simulink model "sim_finale_1"  (R2024a)
settings: Solver=FixedStepAuto  StartTime=0.0  StopTime=40  FixedStep=0.001  RelTol=1e-3
undefined symbols (not defined in the file): A_p, A_y, aero_variabile_con_M, Attitude_0, Attitude_riferimento, b, B_p, B_pz, B_y, B_yz, C_A, C_l, C_m_alpha, C_N_alpha, C_p, C_y, conv_cost_distE, conv_cost_distN, conv_cost_eta, conv_cost_p, conv_cost_y, conv_cost_zeta, D_pz, D_yz, Env, F, G_wE, G_wN, G_xp, G_xy, I_sp, inertia_p, inertia_s, inertia_tot, L, m_p, m_s, m_tot, MIL, Moderate, P_p, P_y, R, r_cp_cm, r_nozzle_cm, S_rif, spinta_variabile, T_c, T_r, v_0, V_r, VelocitB_riferimento, w_0
libraries: cstblocks x16, simulink_extras x5, slpidlib x4, simulink x3, aerolibasang x3, aerolibwind2 x3, matrix_library x2, shared6dof x2, aerolibatmos2 x2, aerolibutil x1, aerolibanim x1
(part 2 of 2)

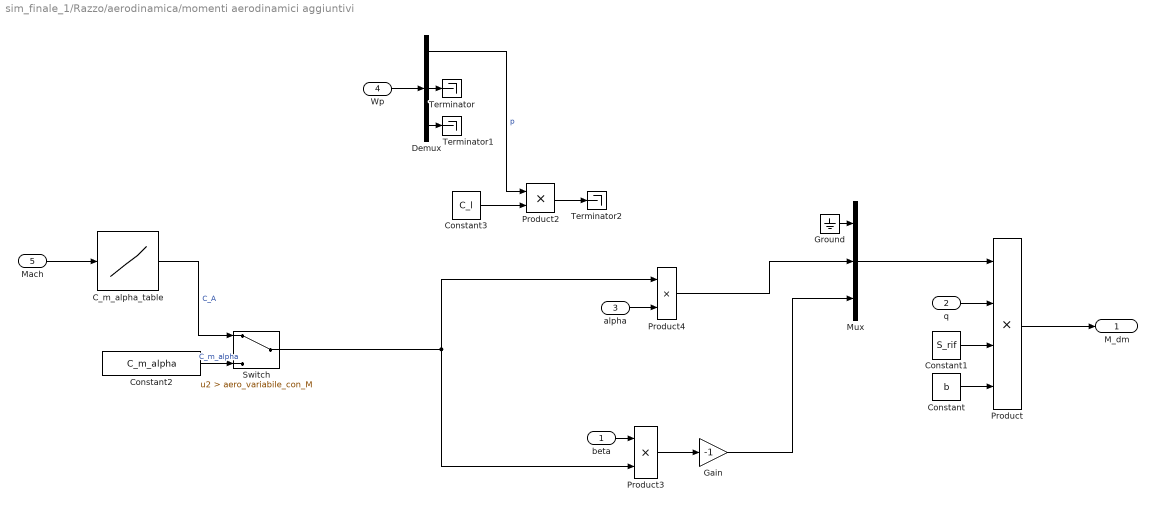
== system sim_finale_1/Razzo/aerodinamica/momenti aerodinamici aggiuntivi ==
  beta : Inport
  q : Inport  Port=2
  alpha : Inport  Port=3
  Wp : Inport  Port=4
  Mach : Inport  Port=5
  C_m_alpha_table : Lookup_n-D  NumberOfTableDimensions=1  BreakpointsForDimension1=[0;0.7;0.95;1.35;1.5;1.95;2.8;3;3.5;4;4.5;5]  Table=[1.75;2;2.05;2.2;2.25;2.5;3.4;3.45;3.6;4.05;4.15;5.15]  InternalRulePriority=Speed  RndMeth=Simplest
  Constant : Constant  Value=b
  Constant1 : Constant  Value=S_rif
  Constant2 : Constant  Value=C_m_alpha
  Constant3 : Constant  Value=C_l
  Demux : Demux  Outputs=3
  Gain : Gain  Gain=-1
  Ground : Ground
  Mux : Mux  Inputs=3
  Product : Product  Inputs=4
  Product2 : Product
  Product3 : Product
  Product4 : Product
  Switch : Switch  Criteria=u2 > Threshold  Threshold=aero_variabile_con_M  SaturateOnIntegerOverflow=off  InputSameDT=off
  Terminator : Terminator
  Terminator1 : Terminator
  Terminator2 : Terminator
  M_dm : Outport
  wires:
  Mux/1 -> Product/1
  Product/1 -> M_dm/1
  Wp/1 -> Demux/1
  Demux/1 -> Product2/1  "p"
  Constant3/1 -> Product2/2
  Product3/1 -> Gain/1
  Constant1/1 -> Product/3
  Constant/1 -> Product/4
  q/1 -> Product/2
  Gain/1 -> Mux/3
  Product4/1 -> Mux/2
  alpha/1 -> Product4/2
  beta/1 -> Product3/1
  Demux/2 -> Terminator/1
  Demux/3 -> Terminator1/1
  Product2/1 -> Terminator2/1
  Ground/1 -> Mux/1
  Switch/1 -> Product4/1, Product3/2
  Constant2/1 -> Switch/3  "C_m_alpha"
  C_m_alpha_table/1 -> Switch/1  "C_A"
  Mach/1 -> C_m_alpha_table/1

== system sim_finale_1/Razzo/massa/massa costante ==
  Constant : Constant  Value=m_tot
  Constant1 : Constant  Value=m_p
  Constant6 : Constant  Value=inertia_tot
  Ground : Ground
  I : Outport
  I_dot : Outport  Port=2
  m : Outport  Port=3
  tag scope: m_p=global
  wires:
  Constant/1 -> m/1
  Ground/1 -> I_dot/1
  Constant6/1 -> I/1
  Constant1/1 -> [m_p]

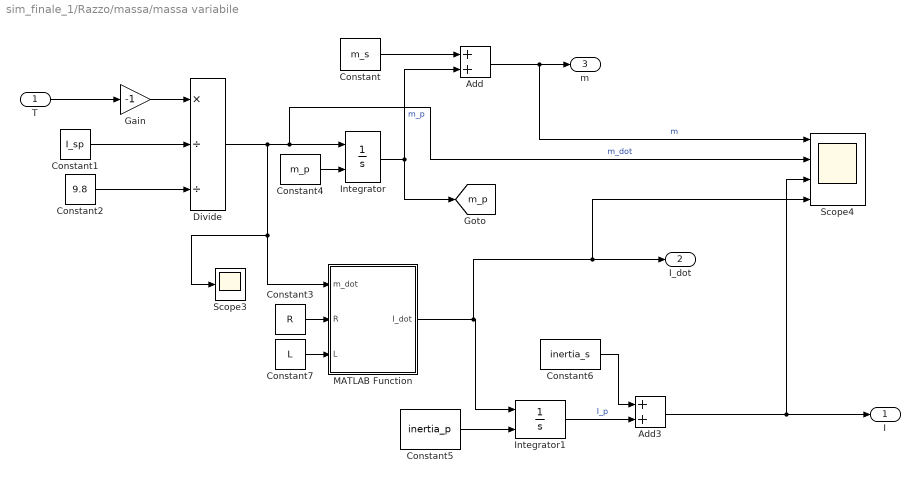
== system sim_finale_1/Razzo/massa/massa variabile ==
  T : Inport
  Add : Sum
  Add3 : Sum
  Constant : Constant  Value=m_s
  Constant1 : Constant  Value=I_sp
  Constant2 : Constant  Value=9.8
  Constant3 : Constant  Value=R
  Constant4 : Constant  Value=m_p
  Constant5 : Constant  Value=inertia_p
  Constant6 : Constant  Value=inertia_s
  Constant7 : Constant  Value=L
  Divide : Product  Inputs=*//
  Gain : Gain  Gain=-1
  Integrator : Integrator  InitialConditionSource=external  LimitOutput=on  LowerSaturationLimit=0
  Integrator1 : Integrator  InitialConditionSource=external  InitialCondition=inertia_p  LimitOutput=on  LowerSaturationLimit=zeros(3)
  MATLAB Function : MATLAB Function  TreatAsAtomicUnit=on
  Scope3 : Scope
  Scope4 : Scope  NumInputPorts=4
  I : Outport
  I_dot : Outport  Port=2
  m : Outport  Port=3
  tag scope: m_p=global
  wires:
  Constant1/1 -> Divide/2
  Constant7/1 -> MATLAB Function/3(L)
  Integrator/1 -> [m_p], Add/2  "m_p"
  Add3/1 -> I/1, Scope4/3
  Constant6/1 -> Add3/1
  Gain/1 -> Divide/1
  Constant4/1 -> Integrator/2
  Constant3/1 -> MATLAB Function/2(R)
  T/1 -> Gain/1
  Add/1 -> Scope4/1, m/1  "m"
  Constant5/1 -> Integrator1/2
  Constant2/1 -> Divide/3
  Constant/1 -> Add/1
  Divide/1 -> Scope3/1, MATLAB Function/1(m_dot), Scope4/2, Integrator/1  "m_dot"
  Integrator1/1 -> Add3/2  "I_p"
  MATLAB Function/1(I_dot) -> Scope4/4, I_dot/1, Integrator1/1

== system sim_finale_1/Variant Subsystem/meno reale/Ambiente ==
  BusElementIn : Inport  PortName=State  Element=Xe
  Atmosfera e gravità : Subsystem  Variant=on
  Demux : Demux  Outputs=3
  Scope : Scope  NumInputPorts=3
  Terminator : Terminator
  Terminator1 : Terminator
  Variant Subsystem : Subsystem  Variant=on
  Bus Element Out : Outport  PortName=Environment  Element=AirDensity
  BusElementOut : Outport  PortName=Environment  Element=SpeedOfSound
  BusElementOut1 : Outport  PortName=Environment  Element=Gravity
  BusElementOut2 : Outport  PortName=Environment  Element=Wind
  BusElementOut3 : Outport  PortName=Environment  Element=Temperature
  wires:
  Demux/1 -> Variant Subsystem/1(Heigh), Atmosfera e gravità/1(Height)  "h"
  Atmosfera e gravità/2(Speed of Sound) -> BusElementOut/1
  Atmosfera e gravità/4(Gravity) -> Scope/1, BusElementOut1/1
  Atmosfera e gravità/1(Temperature) -> BusElementOut3/1
  Variant Subsystem/1(WInd) -> Scope/3, BusElementOut2/1
  BusElementIn/1 -> Demux/1
  Demux/2 -> Terminator/1
  Demux/3 -> Terminator1/1
  Atmosfera e gravità/3(Air Density) -> Scope/2, Bus Element Out/1

== system sim_finale_1/Variant Subsystem/reale/Ambiente1 ==
  BusElementIn : Inport  PortName=State  Element=Xe
  BusElementIn1 : Inport  PortName=State  Element=DCM
  BusElementIn2 : Inport  PortName=State  Element=Vb
  Demux : Demux  Outputs=3
  Scope : Scope  NumInputPorts=3
  Subsystem : Subsystem
  Terminator : Terminator
  Terminator1 : Terminator
  Bus Element Out : Outport  PortName=Environment  Element=AirDensity
  BusElementOut : Outport  PortName=Environment  Element=SpeedOfSound
  BusElementOut1 : Outport  PortName=Environment  Element=Gravity
  BusElementOut2 : Outport  PortName=Environment  Element=Wind
  wires:
  Demux/1 -> Subsystem/3(Height)  "h"
  Subsystem/2(Speed of Sound) -> BusElementOut/1, Scope/3  "a"
  Subsystem/4(Gravity) -> BusElementOut1/1, Scope/1  "g"
  BusElementIn/1 -> Demux/1
  Demux/2 -> Terminator/1
  Demux/3 -> Terminator1/1
  Subsystem/3(Air Density) -> Bus Element Out/1, Scope/2  "rho"
  BusElementIn1/1 -> Subsystem/1(DCM)
  BusElementIn2/1 -> Subsystem/2(Vb)
  Subsystem/1(Wind) -> BusElementOut2/1

== system sim_finale_1/Razzo/Subsystem/Equazioni del moto/Eq. massa costante ==
  F_xyz : Inport
  M_xyz : Inport  Port=2
  6DOF (Euler Angles) : shared6dof/6DOF (Euler Angles)  units=Metric (MKS)  mtype=Fixed  rep=Euler Angles  xme_0=x_0  Vm_0=v_0  eul_0=Attitude_0  pm_0=w_0  mass_0=m_tot  mass_e=0.5  mass_f=2.0  inertia=inertia_tot  inertia_e=eye(3)  inertia_f=2*eye(3)  k_quat=1.0  vre_flag=on  abi_flag=on  aMode=0  xme_statename=''  Vm_statename=''  eul_statename=''  quat_statename=''  pm_statename=''  mass_statename=''
  Ve : Outport
  Xe : Outport  Port=2
  Attitude : Outport  Port=3
  DCM : Outport  Port=4
  Vb : Outport  Port=5
  Wb : Outport  Port=6
  Wb_dot : Outport  Port=7
  Ab : Outport  Port=8
  Ae : Outport  Port=9
  wires:
  6DOF (Euler Angles)/4 -> DCM/1
  F_xyz/1 -> 6DOF (Euler Angles)/1
  M_xyz/1 -> 6DOF (Euler Angles)/2
  6DOF (Euler Angles)/1 -> Ve/1
  6DOF (Euler Angles)/2 -> Xe/1
  6DOF (Euler Angles)/3 -> Attitude/1
  6DOF (Euler Angles)/5 -> Vb/1  "v_b"
  6DOF (Euler Angles)/6 -> Wb/1
  6DOF (Euler Angles)/7 -> Wb_dot/1
  6DOF (Euler Angles)/8 -> Ab/1
  6DOF (Euler Angles)/9 -> Ae/1

== system sim_finale_1/Razzo/Subsystem/Equazioni del moto/Eq. massa variabile ==
  F_xyz : Inport
  M_xyz : Inport  Port=2
  m : Inport  Port=3
  dI/dt : Inport  Port=4
  I : Inport  Port=5
  Custom Variable Mass 6DOF (Euler Angles) : shared6dof/6DOF (Euler Angles)  units=Metric (MKS)  mtype=Custom Variable  rep=Euler Angles  xme_0=x_0  Vm_0=v_0  eul_0=Attitude_0  pm_0=w_0  mass_0=1.0  mass_e=0.5  mass_f=2.0  inertia=eye(3)  inertia_e=eye(3)  inertia_f=2*eye(3)  k_quat=1.0  vre_flag=off  abi_flag=on  aMode=0  xme_statename=''  Vm_statename=''  eul_statename=''  quat_statename=''  pm_statename=''  mass_statename=''
      settings: LibrarySourceBlock=aerolib6dof2/Custom Variable Mass 6DOF (Euler Angles)
  Ve : Outport
  Xe : Outport  Port=2
  Attitude : Outport  Port=3
  DCM : Outport  Port=4
  Vb : Outport  Port=5
  Wb : Outport  Port=6
  Wb_dot : Outport  Port=7
  Ab : Outport  Port=8
  Ae : Outport  Port=9
  wires:
  F_xyz/1 -> Custom Variable Mass 6DOF (Euler Angles)/1
  M_xyz/1 -> Custom Variable Mass 6DOF (Euler Angles)/2
  m/1 -> Custom Variable Mass 6DOF (Euler Angles)/3
  dI/dt/1 -> Custom Variable Mass 6DOF (Euler Angles)/4
  I/1 -> Custom Variable Mass 6DOF (Euler Angles)/5
  Custom Variable Mass 6DOF (Euler Angles)/1 -> Ve/1
  Custom Variable Mass 6DOF (Euler Angles)/2 -> Xe/1
  Custom Variable Mass 6DOF (Euler Angles)/4 -> DCM/1
  Custom Variable Mass 6DOF (Euler Angles)/9 -> Ae/1
  Custom Variable Mass 6DOF (Euler Angles)/3 -> Attitude/1
  Custom Variable Mass 6DOF (Euler Angles)/5 -> Vb/1  "v_b"
  Custom Variable Mass 6DOF (Euler Angles)/6 -> Wb/1
  Custom Variable Mass 6DOF (Euler Angles)/8 -> Ab/1
  Custom Variable Mass 6DOF (Euler Angles)/7 -> Wb_dot/1

== system sim_finale_1/Razzo/aerodinamica/Calcolo F_a e M_a dovuto a F_a in X_a/C_A C_N_alpha ==
  Mach : Inport
  C_A C_N costanti : Subsystem  VariantControl=aero_variabile_con_M == false
  C_A e C_N variabili : Subsystem  VariantControl=aero_variabile_con_M == true
  C_A : Outport
  C_N_alpha : Outport  Port=2

== system sim_finale_1/Variant Subsystem/meno reale/Ambiente/Atmosfera e gravità ==
  Height : Inport
  Env costante : Subsystem  VariantControl="env_variabile  == false"
  Env variabile : Subsystem  VariantControl=env_variabile == true
  Temperature : Outport
  Speed of Sound : Outport  Port=2
  Air Density : Outport  Port=3
  Gravity : Outport  Port=4

== system sim_finale_1/Variant Subsystem/meno reale/Ambiente/Variant Subsystem ==
  note: 1) Add Subsystem or Model blocks as valid variant choices.
      | 2) You cannot connect blocks at this level. At simulation, connectivity is automatically
      | determined, based on the active variant and port name matching.
  Heigh : Inport
  cost Wind : Subsystem  VariantControl=dist_agg==false
  sin Wind : Subsystem  VariantControl=dist_agg==true
  WInd : Outport

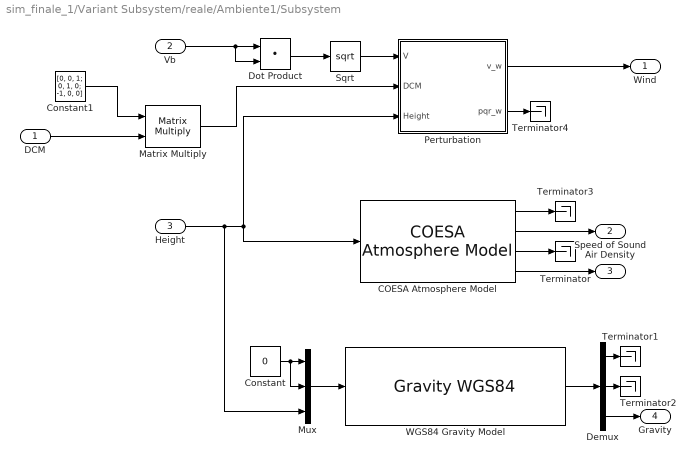
== system sim_finale_1/Variant Subsystem/reale/Ambiente1/Subsystem ==
  DCM : Inport
  Vb : Inport  Port=2
  Height : Inport  Port=3
  COESA Atmosphere Model : aerolibatmos2/COESA Atmosphere Model  units=Metric (MKS)  spec=1976 COESA-extended U.S. Standard Atmosphere  model=Profile  profile_var=High temperature  profile_percent=1%  profile_alt=5 km (16404 ft)  envelope_var=High temperature  envelope_percent=1%  action=Warning
  Constant : Constant  Value=0
  Constant1 : Constant  Value=[0, 0, 1; 0, 1, 0; -1, 0, 0]
  Demux : Demux  Outputs=3
  Dot Product : DotProduct  OutDataTypeStr=Inherit: Inherit via internal rule
  Matrix Multiply : Product  Multiplication=Matrix(*)
  Mux : Mux  Inputs=3
  Perturbation : Subsystem
  Sqrt : Sqrt
  Terminator{,1..4} (5 alike) : Terminator
  "WGS84 Gravity Model  " : GravityWGS84  model=WGS84 Exact  action=None
  Wind : Outport
  Speed of Sound : Outport  Port=2
  Air Density : Outport  Port=3
  Gravity : Outport  Port=4
  wires:
  COESA Atmosphere Model/3 -> Terminator/1
  Height/1 -> COESA Atmosphere Model/1, Perturbation/3(Height), Mux/3
  Perturbation/1(v_w) -> Wind/1
  COESA Atmosphere Model/1 -> Terminator3/1
  Demux/1 -> Terminator1/1
  COESA Atmosphere Model/4 -> Air Density/1
  Demux/2 -> Terminator2/1
  Demux/3 -> Gravity/1
  Dot Product/1 -> Sqrt/1
  Matrix Multiply/1 -> Perturbation/2(DCM)
  Vb/1 -> Dot Product/2, Dot Product/1
  Sqrt/1 -> Perturbation/1(V)
  Constant1/1 -> Matrix Multiply/1
  COESA Atmosphere Model/2 -> Speed of Sound/1
  DCM/1 -> Matrix Multiply/2
  "WGS84 Gravity Model  "/1 -> Demux/1
  Mux/1 -> "WGS84 Gravity Model  "/1
  Constant/1 -> Mux/2, Mux/1
  Perturbation/2(pqr_w) -> Terminator4/1

== system sim_finale_1/Razzo/aerodinamica/Calcolo F_a e M_a dovuto a F_a in X_a/C_A C_N_alpha/C_A C_N costanti ==
  Mach : Inport
  Constant : Constant  Value=C_A
  Constant1 : Constant  Value=C_N_alpha
  Terminator : Terminator
  C_A : Outport
  C_N_alpha : Outport  Port=2
  wires:
  Constant1/1 -> C_N_alpha/1
  Constant/1 -> C_A/1
  Mach/1 -> Terminator/1

== system sim_finale_1/Razzo/aerodinamica/Calcolo F_a e M_a dovuto a F_a in X_a/C_A C_N_alpha/C_A e C_N variabili ==
  Mach : Inport
  C_A_lookup_table : Lookup_n-D  NumberOfTableDimensions=1  BreakpointsForDimension1=[0.2;0.5;0.7;0.9;1.08;1.3;1.5;1.9;2.7;4.3;5]  Table=[0;0.82;1.1;1.5;2.28;2.43;2.48;2.35;1.9;1.3;1.1]  InternalRulePriority=Speed  RndMeth=Simplest
  C_N_AoA_lookup_table : Lookup_n-D  NumberOfTableDimensions=1  BreakpointsForDimension1=[0;0.75;1;1.5;2;2.7;3;3.4;4;4.4;5]  Table=[0.123;0.123;0.14;0.147;0.143;0.18;0.18;0.19;0.207;0.212;0.26]  InternalRulePriority=Speed  RndMeth=Simplest
  To Workspace : ToWorkspace  VariableName=C_N_alpha  SaveFormat=Timeseries  SampleTime=-1
  To Workspace1 : ToWorkspace  VariableName=C_A  SaveFormat=Timeseries  SampleTime=-1
  C_A : Outport
  C_N_alpha : Outport  Port=2
  wires:
  Mach/1 -> C_N_AoA_lookup_table/1, C_A_lookup_table/1
  C_A_lookup_table/1 -> To Workspace/1, C_A/1  "C_A"
  C_N_AoA_lookup_table/1 -> To Workspace1/1, C_N_alpha/1  "C_A"

== system sim_finale_1/Variant Subsystem/meno reale/Ambiente/Atmosfera e gravità/Env costante ==
  Height : Inport
  Constant : Constant  Value=Env.AirDensity
  Constant1 : Constant  Value=Env.Gravity
  Constant2 : Constant  Value=Env.AirPressure
  Constant3 : Constant  Value=Env.SpeedOfSound
  Constant4 : Constant  Value=Env.Temperature
  Terminator : Terminator
  Terminator1 : Terminator
  Temperature : Outport
  Speed of Sound : Outport  Port=2
  Air Density : Outport  Port=3
  Gravity : Outport  Port=4
  wires:
  Height/1 -> Terminator/1
  Constant4/1 -> Temperature/1
  Constant1/1 -> Gravity/1
  Constant3/1 -> Speed of Sound/1
  Constant/1 -> Air Density/1
  Constant2/1 -> Terminator1/1

== system sim_finale_1/Variant Subsystem/meno reale/Ambiente/Atmosfera e gravità/Env variabile ==
  Height : Inport
  Demux : Demux  Outputs=3
  Ground : Ground
  Ground1 : Ground
  ISA Atmosphere Model : aerolibatmos2/ISA Atmosphere Model  useExtended=on  action=Warning  custom=off  viscosityOut=off  g=9.80665  gamma=1.4  R=287.0531  L=0.0065  h_trop=11000  h_strat=20000  rho0=1.225  P0=101325  T0=288.15  h0=0  S=110.4  Tref=273.15  muref=1.716e-5
  Mux : Mux  Inputs=3
  Terminator : Terminator
  Terminator1 : Terminator
  Terminator2 : Terminator
  "WGS84 Gravity Model  " : GravityWGS84
  Temperature : Outport
  Speed of Sound : Outport  Port=2
  Air Density : Outport  Port=3
  Gravity : Outport  Port=4
  wires:
  Height/1 -> Mux/3, ISA Atmosphere Model/1
  ISA Atmosphere Model/2 -> Speed of Sound/1
  ISA Atmosphere Model/4 -> Air Density/1
  ISA Atmosphere Model/3 -> Terminator/1
  ISA Atmosphere Model/1 -> Temperature/1
  Mux/1 -> "WGS84 Gravity Model  "/1
  Ground/1 -> Mux/1
  Ground1/1 -> Mux/2
  "WGS84 Gravity Model  "/1 -> Demux/1
  Demux/3 -> Gravity/1
  Demux/1 -> Terminator1/1
  Demux/2 -> Terminator2/1

== system sim_finale_1/Variant Subsystem/meno reale/Ambiente/Variant Subsystem/cost Wind ==
  Heigh : Inport
  Scope : Scope
  Step : Step  Time=3  After=Env.WindVelocity  SampleTime=0
  WInd : Outport
  wires:
  Step/1 -> WInd/1, Scope/1  "v_w"

== system sim_finale_1/Variant Subsystem/meno reale/Ambiente/Variant Subsystem/sin Wind ==
  Heigh : Inport
  Clock : Clock
  Clock1 : Clock
  Gain : Gain  Gain=5
  Gain1 : Gain  Gain=15
  Ground : Ground
  Scope : Scope
  Sin : Trigonometry
  Step : Step  After=Env.WindVelocity  SampleTime=0
  Sum : Sum  Inputs=|++
  Switch : Switch  Criteria=u2 > Threshold  Threshold=2  SaturateOnIntegerOverflow=off  InputSameDT=off
  WInd : Outport
  wires:
  Step/1 -> Sum/1
  Sum/1 -> WInd/1, Scope/1  "v_w"
  Clock/1 -> Gain/1  "v_w"
  Gain/1 -> Sin/1
  Clock1/1 -> Switch/2
  Switch/1 -> Sum/2
  Ground/1 -> Switch/3
  Gain1/1 -> Switch/1
  Sin/1 -> Gain1/1

== system sim_finale_1/Variant Subsystem/reale/Ambiente1/Subsystem/Perturbation ==
  V : Inport
  DCM : Inport  Port=2
  Height : Inport  Port=3
  Discrete Wind Gust Model : aerolibwind2/Discrete Wind Gust Model  units=Metric (MKS)  Gx=on  Gy=on  Gz=on  t_0=0  d_m=[120 120 80]  v_m=Gust_amplitude
  Dryden Wind Turbulence Model (Discrete (+q -r)) : aerolibwind2/Dryden Wind Turbulence Model  (Continuous (+q -r))  units=Metric (MKS)  spec=MIL-F-8785C  model=Discrete Dryden (+q -r)  W20=V_w  Wdeg=Wind_direction  TurbProb=10^-3 - Moderate  L_high=533.4  Wingspan=10  ts=0.1  Seed=[23341 23342 23343 23344]  T_on=on
      settings: LibrarySourceBlock=|
      | aerolibwind2/Dryden Wind Turbulence Model
      | (Discrete (+q -r))
  Scope : Scope
  Sum : Sum  Inputs=+++
  Wind Shear Model : aerolibwind2/Wind Shear Model  units=Metric (MKS)  phase=Category C - Terminal Flight Phase  W_20=V_w  Wdeg=Wind_direction
  v_w : Outport
  pqr_w : Outport  Port=2
  wires:
  Sum/1 -> Scope/1, v_w/1
  Dryden Wind Turbulence Model (Discrete (+q -r))/2 -> pqr_w/1
  V/1 -> Dryden Wind Turbulence Model (Discrete (+q -r))/2, Discrete Wind Gust Model/1
  DCM/1 -> Dryden Wind Turbulence Model (Discrete (+q -r))/3, Wind Shear Model/2
  Height/1 -> Dryden Wind Turbulence Model (Discrete (+q -r))/1, Wind Shear Model/1
  Wind Shear Model/1 -> Sum/1
  Dryden Wind Turbulence Model (Discrete (+q -r))/1 -> Sum/2
  Discrete Wind Gust Model/1 -> Sum/3

== matlab function sim_finale_1/Razzo/Motore/MATLAB Function ==
  data: TVC_angles input; R_BN output
function R_BN = fcn(TVC_angles)
zeta = TVC_angles(1);
eta = TVC_angles(2);
R_BN = [    cos(zeta)*cos(eta),    -sin(zeta),     cos(zeta)*sin(eta);
            sin(zeta)*cos(eta),    cos(zeta),      sin(zeta)*sin(eta);
            -sin(eta),             0,              cos(eta);
       ];

== matlab function sim_finale_1/Razzo/massa/massa variabile/MATLAB Function ==
  data: m_dot input; I_dot output; R input; L input
function I_dot = fcn(m_dot, R, L)
k_xx = (R^2)/2;
k_yy_zz = (R^2)/4 + (L^2)/12;
J_p_dot = k_xx * m_dot;
I_p_dot = k_yy_zz * m_dot;
I_dot =   [ J_p_dot,   0,           0;
            0,         I_p_dot,     0;
            0,         0,           I_p_dot;
          ];
